simulink model "seguimiento_consignas_constantes_modelo_no_lineal"  (R2021a)
settings: Solver=VariableStepAuto  StartTime=0.0  StopTime=300  RelTol=1e-3
settings Model: Creator=jmata  LastModifiedBy=jmata

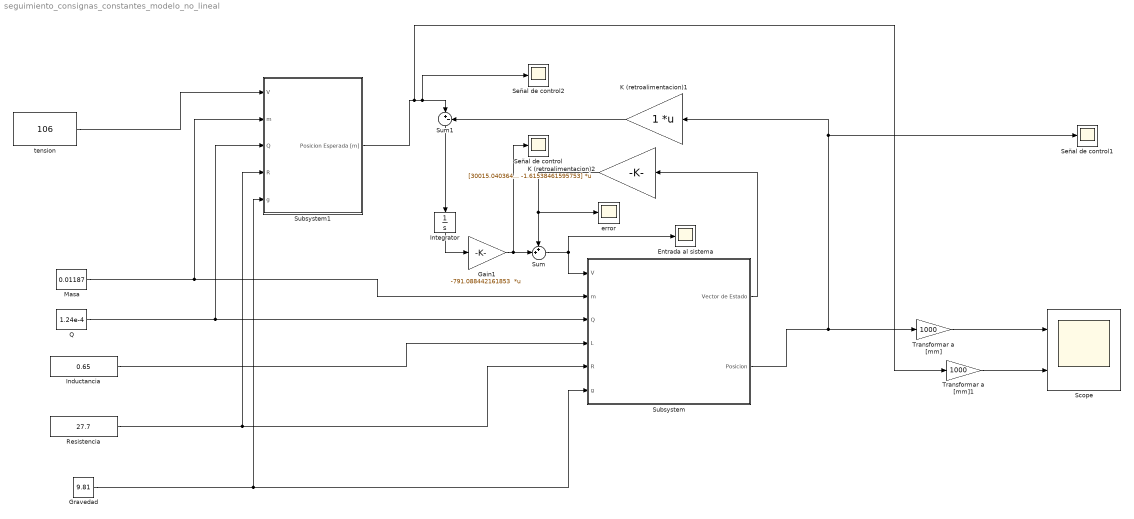
== system seguimiento_consignas_constantes_modelo_no_lineal ==
  Entrada al sistema : Scope
  Gain1 : Gain  Gain=-791.088442161853  Multiplication=Matrix(K*u)
  Gravedad : Constant  Value=9.81
  Inductancia : Constant  Value=0.65
  Integrator : Integrator
  K (retroalimentacion)1 : Gain  Multiplication=Matrix(K*u)
  K (retroalimentacion)2 : Gain  Gain=[30015.0403648094 1205.09300494195 -1.61538461595753]  Multiplication=Matrix(K*u)
  Masa : Constant  Value=0.01187
  Q : Constant  Value=1.24e-4
  Resistencia : Constant  Value=27.7
  Scope : Scope  NumInputPorts=2
  Señal de control : Scope
  Señal de control1 : Scope
  Señal de control2 : Scope
  Subsystem : Subsystem
  Subsystem1 : Subsystem
  Sum : Sum  Inputs=++|
  Sum1 : Sum  Inputs=|+-
  Transformar a [mm] : Gain  Gain=1000
  Transformar a [mm]1 : Gain  Gain=1000
  error : Scope
  tension : Constant  Value=106
  wires:
  Masa/1 -> Subsystem1/2(m), Subsystem/2(m)
  Q/1 -> Subsystem1/3(Q), Subsystem/3(Q)
  Inductancia/1 -> Subsystem/4(L)
  Resistencia/1 -> Subsystem1/4(R), Subsystem/5(R)
  Gravedad/1 -> Subsystem/6(g), Subsystem1/5(g)
  Subsystem/1(Vector de Estado) -> K (retroalimentacion)2/1
  K (retroalimentacion)2/1 -> Sum/1, error/1
  Transformar a [mm]/1 -> Scope/1
  Subsystem/2(Posicion) -> Señal de control1/1, K (retroalimentacion)1/1, Transformar a [mm]/1
  Sum/1 -> Subsystem/1(V), Entrada al sistema/1
  Gain1/1 -> Señal de control/1, Sum/2
  Integrator/1 -> Gain1/1
  Sum1/1 -> Integrator/1
  K (retroalimentacion)1/1 -> Sum1/2
  tension/1 -> Subsystem1/1(V)
  Subsystem1/1("Posicion Esperada [m] ") -> Transformar a [mm]1/1, Señal de control2/1, Sum1/1
  Transformar a [mm]1/1 -> Scope/2

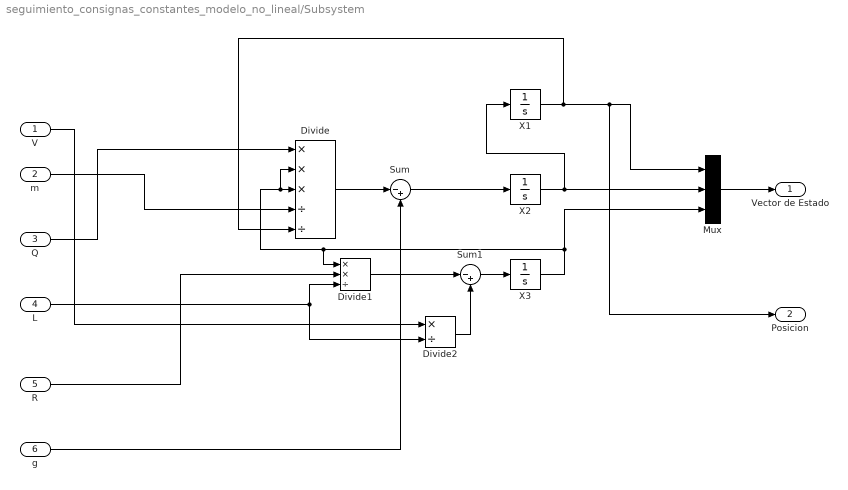
== system seguimiento_consignas_constantes_modelo_no_lineal/Subsystem ==
  V : Inport
  m : Inport  Port=2
  Q : Inport  Port=3
  L : Inport  Port=4
  R : Inport  Port=5
  g : Inport  Port=6
  Divide : Product  Inputs=***//
  Divide1 : Product  Inputs=**/
  Divide2 : Product  Inputs=*/
  Mux : Mux  Inputs=3
  Sum : Sum  Inputs=|-+
  Sum1 : Sum  Inputs=|-+
  X1 : Integrator  InitialCondition=0.00175
  X2 : Integrator
  X3 : Integrator
  Vector de Estado : Outport
  Posicion : Outport  Port=2
  wires:
  Divide/1 -> Sum/1
  Sum/1 -> X2/1
  L/1 -> Divide2/2, Divide1/3
  Sum1/1 -> X3/1
  X3/1 -> Mux/3, Divide1/1, Divide/2, Divide/3
  Divide2/1 -> Sum1/2
  X1/1 -> Posicion/1, Mux/1, Divide/5
  X2/1 -> Mux/2, X1/1
  g/1 -> Sum/2
  Divide1/1 -> Sum1/1
  m/1 -> Divide/4
  Q/1 -> Divide/1
  Mux/1 -> Vector de Estado/1
  R/1 -> Divide1/2
  V/1 -> Divide2/1

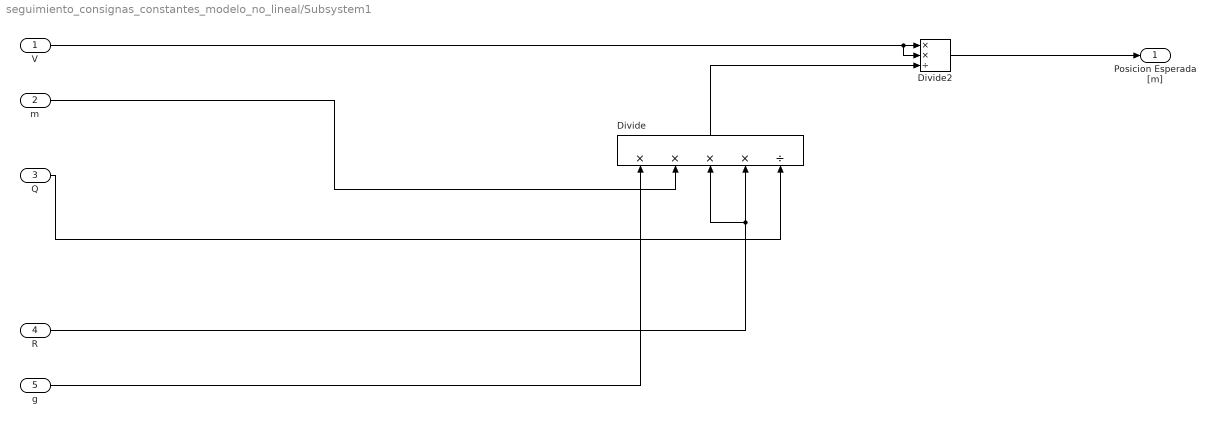
== system seguimiento_consignas_constantes_modelo_no_lineal/Subsystem1 ==
  V : Inport
  m : Inport  Port=2
  Q : Inport  Port=3
  R : Inport  Port=4
  g : Inport  Port=5
  Divide : Product  Inputs=****/
  Divide2 : Product  Inputs=**/
  "Posicion Esperada [m] " : Outport
  wires:
  R/1 -> Divide/3, Divide/4
  Divide/1 -> Divide2/3
  Q/1 -> Divide/5
  m/1 -> Divide/2
  Divide2/1 -> "Posicion Esperada [m] "/1
  g/1 -> Divide/1
  V/1 -> Divide2/2, Divide2/1
